simulink model "Digital_Control"  (R2023a)
settings: Solver=VariableStepAuto  StartTime=0.0  StopTime=80  RelTol=1e-3
values from neighbouring files (symbols this model uses):
  CP = 0.0549    [Digital_Control.m]
  G = c2d(Gs,T,'zoh')    [Digital_Control.m]
  PI_disc = K_linha*tf([1,-K_zero],[1,-1],T)    [Digital_Control.m]
settings Model: Creator=hugo  LastModifiedBy=hugo

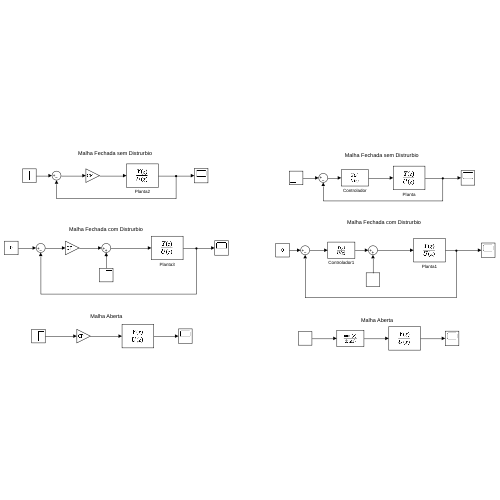
[thumbnail: Simulink's stored preview of the top-level diagram]
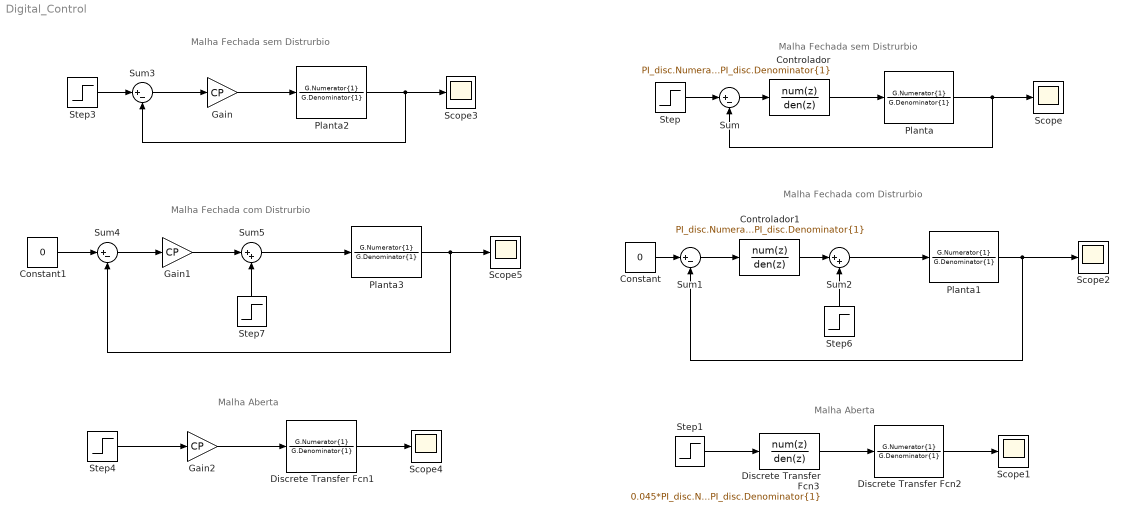
== system Digital_Control ==
  note: Malha Fechada sem Distrurbio
  note: Malha Aberta
  note: Malha Fechada com Distrurbio
  note: Malha Aberta
  note: Malha Fechada sem Distrurbio
  note: Malha Fechada com Distrurbio
  Constant : Constant  Value=0
  Constant1 : Constant  Value=0
  Controlador : DiscreteTransferFcn  Numerator=PI_disc.Numerator{1}  Denominator=PI_disc.Denominator{1}
  Controlador1 : DiscreteTransferFcn  Numerator=PI_disc.Numerator{1}  Denominator=PI_disc.Denominator{1}
  Discrete Transfer Fcn1 : DiscreteTransferFcn  Numerator=G.Numerator{1}  Denominator=G.Denominator{1}
  Discrete Transfer Fcn2 : DiscreteTransferFcn  Numerator=G.Numerator{1}  Denominator=G.Denominator{1}
  Discrete Transfer Fcn3 : DiscreteTransferFcn  Numerator=0.045*PI_disc.Numerator{1}  Denominator=PI_disc.Denominator{1}
  Gain : Gain  Gain=CP
  Gain1 : Gain  Gain=CP
  Gain2 : Gain  Gain=CP
  Planta{,1..3} (4 alike) : DiscreteTransferFcn  Numerator=G.Numerator{1}  Denominator=G.Denominator{1}
  Scope{,1..5} (6 alike) : Scope
  Step{,1,3..4} (4 alike) : Step  Time=0  SampleTime=0.1
  Step6 : Step  Time=5  After=0.1  SampleTime=0.1
  Step7 : Step  Time=2  After=0.1  SampleTime=0.1
  Sum{,1,3..4} (4 alike) : Sum  Inputs=|+-
  Sum2 : Sum  Inputs=|++
  Sum5 : Sum  Inputs=|++
  wires:
  Controlador/1 -> Planta/1
  Planta/1 -> Scope/1, Sum/2
  Sum/1 -> Controlador/1
  Step/1 -> Sum/1
  Discrete Transfer Fcn2/1 -> Scope1/1
  Step1/1 -> Discrete Transfer Fcn3/1
  Discrete Transfer Fcn3/1 -> Discrete Transfer Fcn2/1
  Planta1/1 -> Scope2/1, Sum1/2
  Constant/1 -> Sum1/1
  Sum1/1 -> Controlador1/1
  Planta3/1 -> Scope5/1, Sum4/2
  Constant1/1 -> Sum4/1
  Step4/1 -> Gain2/1
  Step7/1 -> Sum5/2
  Step3/1 -> Sum3/1
  Gain1/1 -> Sum5/1
  Gain/1 -> Planta2/1
  Sum4/1 -> Gain1/1
  Planta2/1 -> Scope3/1, Sum3/2
  Sum3/1 -> Gain/1
  Discrete Transfer Fcn1/1 -> Scope4/1
  Sum5/1 -> Planta3/1
  Gain2/1 -> Discrete Transfer Fcn1/1
  Step6/1 -> Sum2/2
  Controlador1/1 -> Sum2/1
  Sum2/1 -> Planta1/1
